simulink model "lab_exer_mat_2"  (R2015a)
settings: Solver=ode45  StartTime=0.0  StopTime=inf  RelTol=1e-3
InitFcn:
  | CB_Init;
StopFcn:
  | CB_Stop;
values from neighbouring files (symbols this model uses):
  T_Rx = 1    [CB_Init.m]
  T_Tx = 1    [CB_Init.m]
settings Model: Creator=ees1504  LastModifiedBy=tamias
settings OptimizationCC: ExpressionDepthLimit=2147483647
settings DebuggingCC: UnderspecifiedInitializationDetection=Classic  MergeDetectMultiDrivingBlocksExec=none  SolverPrmCheckMsg=warning  StateNameClashWarn=warning
settings GRTTargetCC: CombineOutputUpdateFcns=off  GRTInterface=on

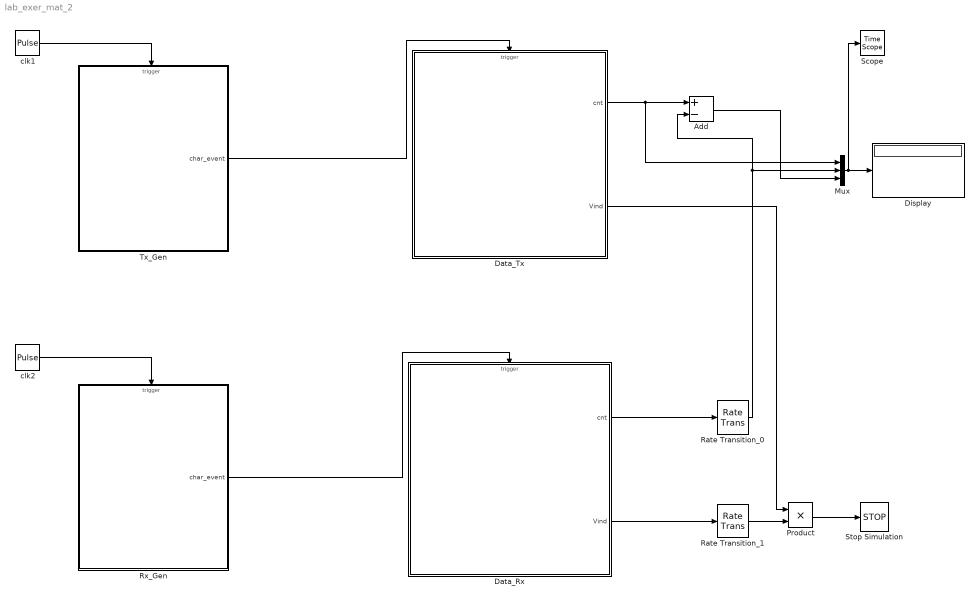
== system lab_exer_mat_2 ==
  Add : Sum  Inputs=+-  AccumDataTypeStr=double  OutDataTypeStr=double
  Data_Rx : Stateflow chart  TreatAsAtomicUnit=on
  Data_Tx : Stateflow chart  TreatAsAtomicUnit=on
  Display : Display
  Mux : Mux  Inputs=3
  Product : Product  RndMeth=Zero
  Rate Transition_0 : RateTransition
  Rate Transition_1 : RateTransition
  Rx_Gen : Stateflow chart  TreatAsAtomicUnit=on
  Scope : TimeScope
  Stop Simulation : Stop
  Tx_Gen : Stateflow chart  TreatAsAtomicUnit=on
  clk1 : DiscretePulseGenerator  PulseType=Time based  Period=T_Tx  PulseWidth=0.5
  clk2 : DiscretePulseGenerator  PulseType=Time based  Period=T_Rx  PulseWidth=0.5
  wires:
  Data_Rx/1(cnt) -> Rate Transition_0/1
  Data_Rx/2(Vind) -> Rate Transition_1/1
  Rate Transition_1/1 -> Product/2
  Product/1 -> Stop Simulation/1
  Data_Tx/1(cnt) -> Add/1, Mux/1
  Data_Tx/2(Vind) -> Product/1
  Mux/1 -> Display/1, Scope/1
  Rate Transition_0/1 -> Add/2, Mux/2
  clk1/1 -> Tx_Gen/Trigger
  clk2/1 -> Rx_Gen/Trigger
  Tx_Gen/1(char_event) -> Data_Tx/Trigger
  Rx_Gen/1(char_event) -> Data_Rx/Trigger
  Add/1 -> Mux/3

== stateflow chart lab_exer_mat_2/Data_Tx ==
  state STOP
    entry: Vind = 1;
  state INIT
    entry: cnt = cnt+1;
  state FULL
  state TRANSMIT
    entry:
    ml.c_buf[ml.Wp+1]= ml.Tx_buf[cnt];
    ml.Wp = ml.mod(ml.Wp+1, ml.buf_size);
  (default) -> INIT : {cnt = 0;Vind=0;}
  INIT -> STOP [order 2] : [cnt==ml.Nc+1]
  TRANSMIT -> INIT
  INIT -> (junction 8) [order 1] : [cnt!=ml.Nc+1]
  (junction 8) -> FULL [order 1] : [ml.Wp == ml.mod(ml.Rp-1, ml.buf_size)]
  (junction 8) -> TRANSMIT [order 2] : [ml.Wp != ml.mod(ml.Rp-1, ml.buf_size)]
  FULL -> (junction 8)
  data: cnt output double; Vind output double
  events: clk input EITHER_EDGE_EVENT

== stateflow chart lab_exer_mat_2/Data_Rx ==
  state STOP
    entry: Vind = 1;
  state INIT
    entry: cnt = cnt+1;
  state EMPTY
  state RECIEVE
    entry:
    ml.Rx_buf[cnt] = ml.c_buf[ml.Rp+1];
    ml.Rp = ml.mod(ml.Rp+1, ml.buf_size);
  (default) -> INIT : {cnt = 0;Vind=0;}
  INIT -> STOP [order 2] : [cnt == ml.Nc+1]
  RECIEVE -> INIT
  INIT -> (junction 4) [order 1] : [cnt != ml.Nc+1]
  (junction 4) -> EMPTY [order 1] : [ml.Wp == ml.Rp]
  (junction 4) -> RECIEVE [order 2] : [ml.Wp != ml.Rp]
  EMPTY -> (junction 4)
  data: cnt output double; Vind output double
  events: clk input EITHER_EDGE_EVENT

== stateflow chart lab_exer_mat_2/Tx_Gen ==
  state C [parallel]
    settings: executionOrder=1
    state UpCounter
      entry: upc = upc + 1;
      during: upc = upc + 1;
      UpCounter -> UpCounter
    (default) -> UpCounter : {upc=0;}
  state D [parallel]
    settings: executionOrder=2
    state S0
      entry: cnt = cnt + 1;
      char_event;
      ml.char_vals[cnt] = ml.randi(ml.Range, 1, 1);
      ml.time_vals[cnt] = upc;
    state S5
    state S4
    state S3
    state S2
    state S1
    (default) -> S0 : {cnt=0;}
    S5 -> S0
    (junction 61) -> S0 [order 2] : [val<=ml.qs[3]]
    S0 -> (junction 53)
    (junction 28) -> S0 [order 1] : [val<=ml.qs[1]]
    (junction 34) -> S0 [order 2] : [val<=ml.qs[2]]
    S4 -> (junction 61) : {val=ml.rand(1);}
    (junction 61) -> S5 [order 1] : [val>ml.qs[3]]
    (junction 53) -> S1
    S3 -> S4
    (junction 34) -> S3 [order 1] : [val>ml.qs[2]]
    (junction 28) -> S2 [order 2] : [val>ml.qs[1]]
    S2 -> (junction 34) : {val=ml.rand(1);}
    S1 -> (junction 28) : {val=ml.rand(1);}
  data: val local double; cnt local double; upc local int32
  events: clk input RISING_EDGE_EVENT; char_event output EITHER_EDGE_EVENT

== stateflow chart lab_exer_mat_2/Rx_Gen ==
  state C [parallel]
    settings: executionOrder=1
    state UpCounter
      entry: upc = upc + 1;
      during: upc = upc + 1;
      UpCounter -> UpCounter
    (default) -> UpCounter : {upc=0;}
  state D [parallel]
    settings: executionOrder=2
    state S0
      entry: cnt = cnt + 1;
      char_event;
      ml.char_vals[cnt] = ml.randi(ml.Range, 1, 1);
      ml.time_vals[cnt] = upc;
    state S5
    state S4
    state S3
    state S2
    state S1
    (default) -> S0 : {cnt=0;}
    S5 -> S0
    (junction 61) -> S0 [order 2] : [val<=ml.qs[3]]
    S0 -> (junction 53)
    (junction 28) -> S0 [order 1] : [val<=ml.qs[1]]
    (junction 34) -> S0 [order 2] : [val<=ml.qs[2]]
    S4 -> (junction 61) : {val=ml.rand(1);}
    (junction 61) -> S5 [order 1] : [val>ml.qs[3]]
    (junction 53) -> S1
    S3 -> S4
    (junction 34) -> S3 [order 1] : [val>ml.qs[2]]
    (junction 28) -> S2 [order 2] : [val>ml.qs[1]]
    S2 -> (junction 34) : {val=ml.rand(1);}
    S1 -> (junction 28) : {val=ml.rand(1);}
  data: val local double; cnt local double; upc local int32
  events: clk input RISING_EDGE_EVENT; char_event output EITHER_EDGE_EVENT
